simulink model "blown_lift_model"  (R2018b)
settings: Solver=ode45  StartTime=0.0  StopTime=100  RelTol=1e-5
model workspace (MAT data in the model file):
  aeroCoeff.CD = [0.115; 0.079; 0.047; 0.031; 0.027; 0.027; 0.029; 0.034; 0.054; 0.089]
  aeroCoeff.CL = [-1.421; -1.092; -0.695; -0.312; -0.132; 0.041; 0.218; 0.402; 0.786; 1.186]
  aeroCoeff.CM = [0.0775; 0.0663; 0.053; 0.0337; 0.0217; 0.0073; -0.009; -0.0263; -0.0632; -0.1235]
  aeroCoeff.CD_el = [0.0046  0.0029  0  -0.0009  -0.0008; 0.0039  0.0024  0  -0.0005  -0.0001; 0.0034  0.002  0  0  0.0005; 0.0028  0.0016  0  0.0004  0.0011; 0.0025  0.0014  0  0.0006  0.0014; 0.0022  0.0012  0  0.0008  0.0016; 0.0019  0.001  0  0.001  0.0019; 0.0016  0.0008  0  0.0012  0.0022; 0.001  0.0003  0  0.0016  0.0028; 0.0004  -0.0001  0  0.0021  0.0034]
  aeroCoeff.CL_el = [-0.051; -0.038; 0; 0.038; 0.052]
  aeroCoeff.CM_el = [0.0842; 0.0601; -0.0001; -0.0601; -0.0843]
  aeroCoeff.Xcp = [-0.055; -0.061; -0.076; -0.108; -0.164; 0.177; -0.041; -0.065; -0.08; -0.105]
  aeroCoeff.Mach_vec = [0.1 0.2 0.3 0.35]
  aeroCoeff.alpha_vec = [-16 -12 -8 -4 -2 0 2 4 8 12]
  aeroCoeff.def_vec = [-20 -10 0 10 20]
  environment.T0 = 275.15
  environment.a = 332.529
  environment.P0 = 79495.2
  environment.rho0 = 1.00649
  environment.vel_wind = [-2; 0; -0.1]
  environment.omega_wind = [0; 0; 0]
  environment.grav = [0 0 9.80665]
  initCond.alt0 = 2000
  initCond.x0 = [0 -2000]
  initCond.v0 = 93.1048
  initCond.alpha0 = 0.017092
  initCond.theta0 = 0.017092
  initCond.q0 = 0
  vehicle.Sref = 20.9775
  vehicle.cbar = 1.7526
  vehicle.bref = 12.54
  vehicle.CG = [0 0 0]
  vehicle.inertia_yy = 6928.93
  vehicle.acMass = 1299.214
  vehicle.Thrust = 2512.574
  vehicle.elevator_max = 20
  vehicle.elevator_min = -20
libraries: aerolibasang x3, shared3dof x1, sharedtransform x1
settings Model: Creator=Jacob  LastModifiedBy=william
settings SolverCC: MinimalZcImpactIntegration=on
settings DataIOCC: SaveFormat=Array
settings OptimizationCC: EnhancedBackFolding=on  StrengthReduction=on  InitFltsAndDblsToZero=on  DifferentSizesBufferReuse=on
settings DebuggingCC: WriteAfterWriteMsg=DisableAll  AlgebraicLoopMsg=none  FcnCallInpInsideContextMsg=warning  UnconnectedInputMsg=none  UnconnectedOutputMsg=none  UnconnectedLineMsg=none  UniqueDataStoreMsg=error  StateNameClashWarn=warning  LibraryContextMissingDiagnostic=none  StrictBusMsg=ErrorOnBusTreatedAsVector  SFUnexpectedBacktrackingDiag=warning  SFNoUnconditionalDefaultTransitionDiag=warning  SFExecutionAtInitializationDiag=none
settings ModelReferenceCC: PropagateSignalLabelsOutOfModel=off
settings SFSimCC: SimUseLocalCustomCode=off
settings RTWCC: RTWUseLocalCustomCode=off
settings CodeAppCC: StateflowObjectComments=on

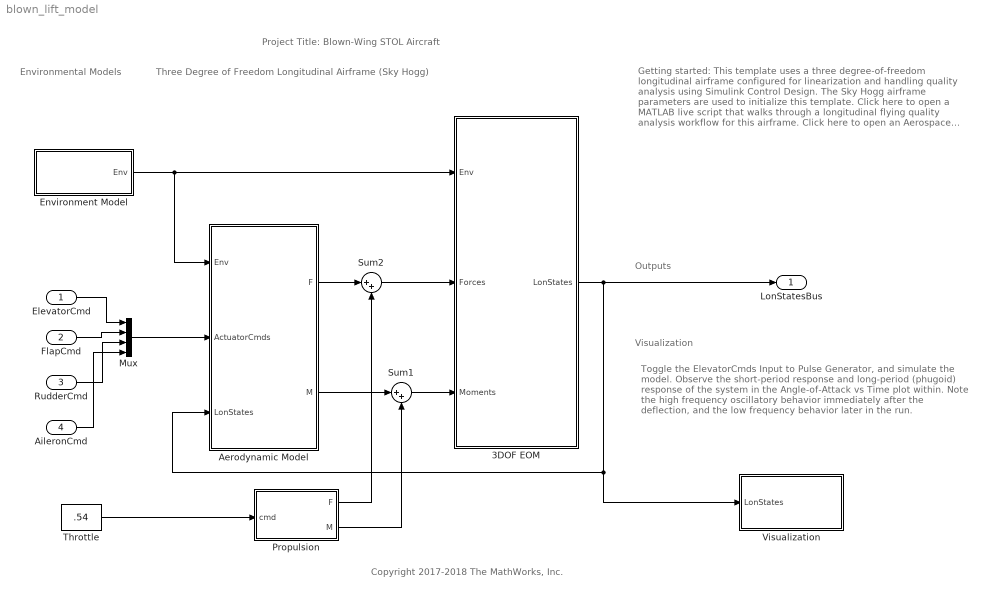
== system blown_lift_model ==
  note: Project Title: Blown-Wing STOL Aircraft
  note: Copyright 2017-2018 The MathWorks, Inc.
  note: Three Degree of Freedom Longitudinal Airframe (Sky Hogg)
  note: Environmental Models
  note: Toggle the ElevatorCmds Input to Pulse Generator, and simulate the model. Observe the short-period response and long-period (phugoid) response of the system in the Angle-of-Attack vs Time plot within. Note the high frequency oscillatory behavior immediately after the deflection, and the low frequency behavior later in the run.
  note: Visualization
  note: Outputs
  note: Getting started:
      | This template uses a three degree-of-freedom longitudinal airframe configured for linearization and handling quality analysis using Simulink Control Design. The Sky Hogg airframe parameters are used to initialize this template.
      |
      | Click here to open a MATLAB live script that walks through a longitudinal flying quality analysis workflow for this airframe.
      |
      | Click here to open an Aerospace Blockset Flight Control Analysis template that can be customized to perform flying quality analysis on your airframe model.
  ElevatorCmd : Inport
  FlapCmd : Inport  Port=2
  RudderCmd : Inport  Port=3
  AileronCmd : Inport  Port=4
  3DOF EOM : Subsystem  VariantControl=eom3DOF
  Aerodynamic Model : Subsystem  VariantControl=aeroCONST
  Environment Model : Subsystem  mask(Constant Environment Model){To=environment.T0, a=environment.a, Po=environment.P0, AirDensity=environment.rho0, ugvgwg=environment.vel_wind, pgqgrg=environment.omega_wind, g=environment.grav}
      mask prompts: To "Constant Temperature (K):"; a "Constant Speed of Sound (m/s):"; Po "Constant Pressure (Pa):"; AirDensity "Constant Air Density (kg/m^3):"; ugvgwg "Constant Wind Velocity [ug vg wg] (m/s):"; pgqgrg "Constant Wind Angular Rates [pg qg rg] (rad/s):"; g "Constant Gravitational Acceleration (m/s^2):"
      mask Help: helpview(fullfile(docroot,'toolbox','aeroblks','aeroblks.map'), 'environment1');
      mask TypeOptions To: Constant Atmosphere/To
      mask TypeOptions a: Constant Atmosphere/a
      mask TypeOptions Po: Constant Atmosphere/Po
      mask TypeOptions AirDensity: Constant Atmosphere/AirDensity
      mask TypeOptions ugvgwg: Constant Wind/ugvgwg
      mask TypeOptions pgqgrg: Constant Wind/pgqgrg
      mask TypeOptions g: Constant Gravity/g
      mask DialogControl Container4 Prompt: Atmospheric Model
      mask DialogControl Container6 Prompt: Wind Model
      mask DialogControl Container8 Prompt: Gravity Model
      mask Display:
      | image('aeroenvironment.bmp','center')
      | port_label('output',1,'Env')
  Mux : Mux
  Propulsion : Subsystem
      settings: RTWSystemCode=Inline
  Sum1 : Sum  Inputs=|++  SaturateOnIntegerOverflow=on  InputSameDT=on  OutDataTypeStr=Inherit: Same as first input
  Sum2 : Sum  Inputs=|++  SaturateOnIntegerOverflow=on  InputSameDT=on  OutDataTypeStr=Inherit: Same as first input
  Throttle : Constant  Value=.54
  Visualization : Subsystem
  LonStatesBus : Outport
  wires:
  3DOF EOM/1(LonStates) -> LonStatesBus/1, Visualization/1(LonStates), Aerodynamic Model/3(LonStates)
  Sum2/1 -> 3DOF EOM/2(Forces)
  Propulsion/2(M) -> Sum1/2
  Propulsion/1(F) -> Sum2/2
  Throttle/1 -> Propulsion/1(cmd)
  Sum1/1 -> 3DOF EOM/3(Moments)
  Aerodynamic Model/1(F) -> Sum2/1
  Aerodynamic Model/2(" M") -> Sum1/1
  Environment Model/1(Env) -> 3DOF EOM/1(Env), Aerodynamic Model/1(Env)
  ElevatorCmd/1 -> Mux/1
  FlapCmd/1 -> Mux/2
  RudderCmd/1 -> Mux/3
  AileronCmd/1 -> Mux/4
  Mux/1 -> Aerodynamic Model/2(ActuatorCmds)

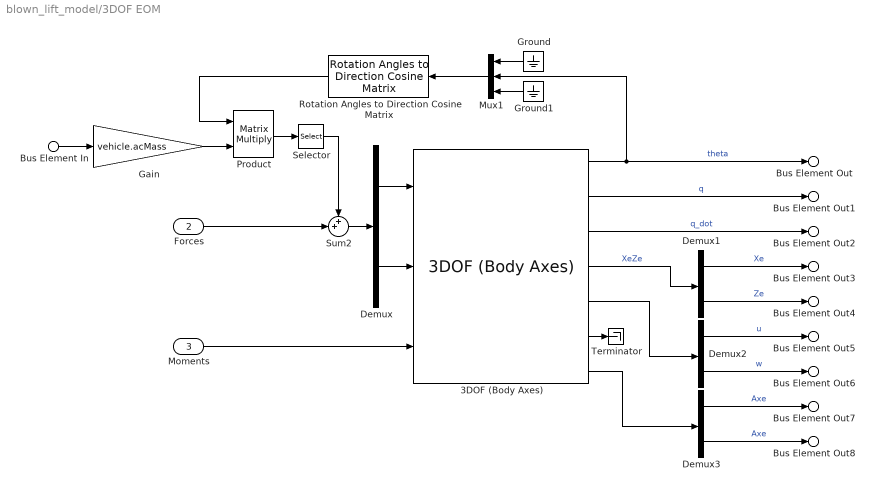
== system blown_lift_model/3DOF EOM ==
  Bus Element In : Inport  PortName=Env  Element=g
  Forces : Inport  Port=2
  Moments : Inport  Port=3
  3DOF (Body Axes) : shared3dof/3DOF (Body Axes)  units=Metric (MKS)  mtype=Fixed  v_ini=initCond.v0  theta_ini=initCond.theta0  alpha_ini=initCond.alpha0  pos_ini=initCond.x0  q_ini=initCond.q0  mass=vehicle.acMass  mass_e=0.5  mass_f=3.0  Iyy=vehicle.inertia_yy  Iyy_e=0.5  Iyy_f=3.0  g_in=Internal  g=0  vre_flag=on  abi_flag=on  aMode=0  vel_statename={'u', 'w'}  theta_statename='theta'  pos_statename={'Xe', 'Ze'}  q_statename='q'  mass_statename=''
      settings: SourceProductName=Aerospace Blockset  SourceProductBaseCode=AE
  Demux{,1..3} (4 alike) : Demux  Outputs=2
  Gain : Gain  Gain=vehicle.acMass
  Ground : Ground
  Ground1 : Ground
  Mux1 : Mux  Inputs=3
  Product : Product  Multiplication=Matrix(*)
  Rotation Angles to Direction Cosine Matrix : sharedtransform/Rotation Angles to Direction Cosine Matrix  rotationOrder=ZYX  aMode=aMode
      settings: SourceProductBaseCode=AE
  Selector : Selector  InputPortWidth=3  IndexOptions=Index vector (dialog)  Indices=[1 3]  OutputSizes=1
  Sum2 : Sum  Inputs=++|  SaturateOnIntegerOverflow=on  InputSameDT=on  OutDataTypeStr=Inherit: Same as first input
  Terminator : Terminator
  Bus Element Out : Outport  PortName=LonStates  Element=theta
  Bus Element Out1 : Outport  PortName=LonStates  Element=q
  Bus Element Out2 : Outport  PortName=LonStates  Element=q_dot
  Bus Element Out3 : Outport  PortName=LonStates  Element=Xe
  Bus Element Out4 : Outport  PortName=LonStates  Element=Ze
  Bus Element Out5 : Outport  PortName=LonStates  Element=u
  Bus Element Out6 : Outport  PortName=LonStates  Element=w
  Bus Element Out7 : Outport  PortName=LonStates  Element=Axe
  Bus Element Out8 : Outport  PortName=LonStates  Element=Aze
  wires:
  Demux/2 -> 3DOF (Body Axes)/2
  Demux/1 -> 3DOF (Body Axes)/1
  Sum2/1 -> Demux/1
  Selector/1 -> Sum2/1
  Ground1/1 -> Mux1/3
  Ground/1 -> Mux1/1
  Mux1/1 -> Rotation Angles to Direction Cosine Matrix/1
  Gain/1 -> Product/2
  Rotation Angles to Direction Cosine Matrix/1 -> Product/1
  Product/1 -> Selector/1
  Forces/1 -> Sum2/2
  Bus Element In/1 -> Gain/1
  Moments/1 -> 3DOF (Body Axes)/3
  3DOF (Body Axes)/1 -> Mux1/2, Bus Element Out/1  "theta"
  3DOF (Body Axes)/2 -> Bus Element Out1/1  "q"
  3DOF (Body Axes)/3 -> Bus Element Out2/1  "q_dot"
  3DOF (Body Axes)/4 -> Demux1/1  "XeZe"
  3DOF (Body Axes)/5 -> Demux2/1
  3DOF (Body Axes)/7 -> Demux3/1
  Demux3/1 -> Bus Element Out7/1  "Axe"
  Demux3/2 -> Bus Element Out8/1  "Axe"
  Demux2/2 -> Bus Element Out6/1  "w"
  Demux2/1 -> Bus Element Out5/1  "u"
  Demux1/2 -> Bus Element Out4/1  "Ze"
  Demux1/1 -> Bus Element Out3/1  "Xe"
  3DOF (Body Axes)/6 -> Terminator/1

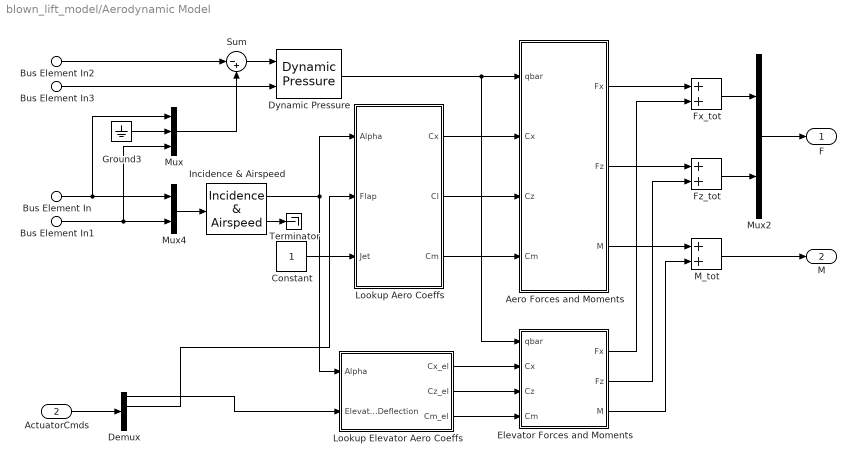
== system blown_lift_model/Aerodynamic Model ==
  Bus Element In2 : Inport  PortName=Env  Element=WindVelocity
  Bus Element In3 : Inport  PortName=Env  Element=AirDensity
  ActuatorCmds : Inport  Port=2
  Bus Element In : Inport  Port=3  PortName=LonStates  Element=u
  Bus Element In1 : Inport  Port=3  PortName=LonStates  Element=w
  Aero Forces and Moments : Subsystem
  Constant : Constant
  Demux : Demux
  Dynamic Pressure : aerolibasang/Dynamic Pressure
  Elevator Forces and Moments : Subsystem
  Fx_tot : Sum  SaturateOnIntegerOverflow=on  InputSameDT=on  OutDataTypeStr=Inherit: Same as first input
  Fz_tot : Sum  SaturateOnIntegerOverflow=on  InputSameDT=on  OutDataTypeStr=Inherit: Same as first input
  Ground3 : Ground
  Incidence & Airspeed : aerolibasang/Incidence  & Airspeed
      settings: SourceProductName=Aerospace Blockset  SourceProductBaseCode=AE
  Lookup Aero Coeffs : Subsystem
  Lookup Elevator Aero Coeffs : Subsystem
  M_tot : Sum  SaturateOnIntegerOverflow=on  InputSameDT=on  OutDataTypeStr=Inherit: Same as first input
  Mux : Mux  Inputs=3
  Mux2 : Mux  Inputs=2
  Mux4 : Mux  Inputs=2
  Sum : Sum  Inputs=|-+
  Terminator : Terminator
  F : Outport
  " M" : Outport  Port=2  Unit=N*m
  wires:
  Bus Element In3/1 -> Dynamic Pressure/2
  Bus Element In2/1 -> Sum/1
  Incidence & Airspeed/2 -> Terminator/1
  Bus Element In/1 -> Mux4/1, Mux/1
  Bus Element In1/1 -> Mux4/2, Mux/3
  Mux2/1 -> F/1
  Mux4/1 -> Incidence & Airspeed/1
  Ground3/1 -> Mux/2
  M_tot/1 -> " M"/1
  Sum/1 -> Dynamic Pressure/1
  Incidence & Airspeed/1 -> Lookup Aero Coeffs/1(Alpha), Lookup Elevator Aero Coeffs/1(Alpha)
  Mux/1 -> Sum/2
  Elevator Forces and Moments/3(M) -> M_tot/2
  Dynamic Pressure/1 -> Elevator Forces and Moments/1(qbar), Aero Forces and Moments/1(qbar)
  Aero Forces and Moments/1(Fx) -> Fx_tot/1
  Aero Forces and Moments/3(M) -> M_tot/1
  Lookup Aero Coeffs/1(Cx) -> Aero Forces and Moments/2(Cx)
  Lookup Aero Coeffs/2(Cl) -> Aero Forces and Moments/3(Cz)
  Lookup Aero Coeffs/3(Cm) -> Aero Forces and Moments/4(Cm)
  Lookup Elevator Aero Coeffs/1(Cx_el) -> Elevator Forces and Moments/2(Cx)
  Lookup Elevator Aero Coeffs/2(Cz_el) -> Elevator Forces and Moments/3(Cz)
  Lookup Elevator Aero Coeffs/3(Cm_el) -> Elevator Forces and Moments/4(Cm)
  Elevator Forces and Moments/1(Fx) -> Fx_tot/2
  Elevator Forces and Moments/2(Fz) -> Fz_tot/2
  Aero Forces and Moments/2(Fz) -> Fz_tot/1
  Fx_tot/1 -> Mux2/1
  Fz_tot/1 -> Mux2/2
  ActuatorCmds/1 -> Demux/1
  Demux/1 -> Lookup Elevator Aero Coeffs/2(Elevator Deflection)
  Demux/2 -> Lookup Aero Coeffs/2(Flap)
  Constant/1 -> Lookup Aero Coeffs/3(Jet)

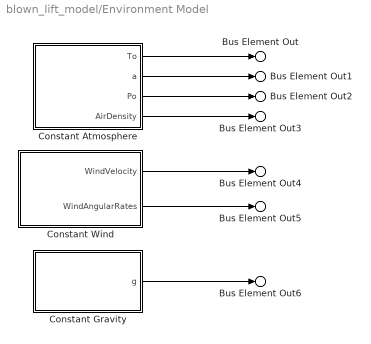
== system blown_lift_model/Environment Model ==
  Constant Atmosphere : Subsystem  VariantControl=atmosCONST  mask(Standard Atmospheric Constants){To=To, a=a, Po=Po, AirDensity=AirDensity}
      mask prompts: To "Constant Temperature (K):"; a "Constant Speed of Sound (m/s):"; Po "Constant Pressure (Pa):"; AirDensity "Constant Air Density (kg/m^3):"
  Constant Gravity : Subsystem  VariantControl=gravCONST  mask(Constant Gravitational Acceleration){g=g}
      mask prompts: g "Constant Gravitational Acceleration (m/s^2):"
  Constant Wind : Subsystem  VariantControl=windCONST  mask(Constant Wind Values){ugvgwg=ugvgwg, pgqgrg=pgqgrg}
      mask prompts: ugvgwg "Constant Wind Velocity (m/s):"; pgqgrg "Constant Wind Angular Rates (rad/s):"
  Bus Element Out : Outport  PortName=Env  Element=To
  Bus Element Out1 : Outport  PortName=Env  Element=a
  Bus Element Out2 : Outport  PortName=Env  Element=Po
  Bus Element Out3 : Outport  PortName=Env  Element=AirDensity
  Bus Element Out4 : Outport  PortName=Env  Element=WindVelocity
  Bus Element Out5 : Outport  PortName=Env  Element=WindAngularRates
  Bus Element Out6 : Outport  PortName=Env  Element=g
  wires:
  Constant Wind/2(WindAngularRates) -> Bus Element Out5/1
  Constant Atmosphere/3(Po) -> Bus Element Out2/1
  Constant Atmosphere/4(AirDensity) -> Bus Element Out3/1
  Constant Atmosphere/1(To) -> Bus Element Out/1
  Constant Wind/1(WindVelocity) -> Bus Element Out4/1
  Constant Atmosphere/2(a) -> Bus Element Out1/1
  Constant Gravity/1(g) -> Bus Element Out6/1

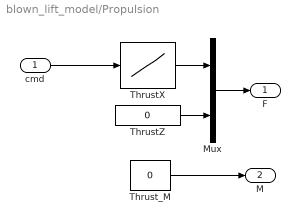
== system blown_lift_model/Propulsion ==
  cmd : Inport
  Mux : Mux  Inputs=2
  ThrustX : Lookup_n-D  NumberOfTableDimensions=1  LookupTableObject=''  BreakpointsForDimension1=(1/6)*(3+([-3:3]))  IndexSearchMethod=Linear search  BeginIndexSearchUsingPreviousIndexResult=on  Table=vehicle.Thrust*(1+tanh([-3:3]))  ExtrapMethod=Clip  InputSameDT=on
  ThrustZ : Constant  Value=0  SampleTime=-1
  Thrust_M : Constant  Value=0  SampleTime=-1
  F : Outport  Unit=N
  M : Outport  Port=2  Unit=N*m
  wires:
  cmd/1 -> ThrustX/1
  Thrust_M/1 -> M/1
  Mux/1 -> F/1
  ThrustZ/1 -> Mux/2
  ThrustX/1 -> Mux/1

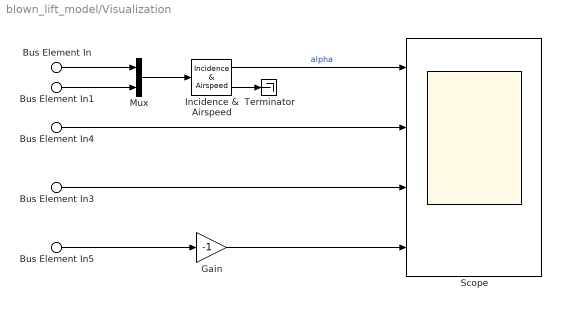
== system blown_lift_model/Visualization ==
  Bus Element In : Inport  PortName=LonStates  Element=u
  Bus Element In1 : Inport  PortName=LonStates  Element=w
  Bus Element In3 : Inport  PortName=LonStates  Element=q
  Bus Element In4 : Inport  PortName=LonStates  Element=theta
  Bus Element In5 : Inport  PortName=LonStates  Element=Ze
  Gain : Gain  Gain=-1
  Incidence & Airspeed : aerolibasang/Incidence  & Airspeed
      settings: SourceProductName=Aerospace Blockset  SourceProductBaseCode=AE
  Mux : Mux  Inputs=2
  Scope : Scope  NumInputPorts=4
  Terminator : Terminator
  wires:
  Gain/1 -> Scope/4
  Bus Element In5/1 -> Gain/1
  Bus Element In4/1 -> Scope/2
  Bus Element In3/1 -> Scope/3
  Mux/1 -> Incidence & Airspeed/1
  Bus Element In1/1 -> Mux/2
  Bus Element In/1 -> Mux/1
  Incidence & Airspeed/2 -> Terminator/1
  Incidence & Airspeed/1 -> Scope/1  "alpha"

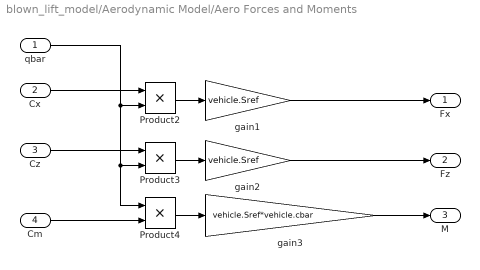
== system blown_lift_model/Aerodynamic Model/Aero Forces and Moments ==
  qbar : Inport
  Cx : Inport  Port=2
  Cz : Inport  Port=3
  Cm : Inport  Port=4
  Product2 : Product  SaturateOnIntegerOverflow=on  InputSameDT=on  OutDataTypeStr=Inherit: Same as first input
  Product3 : Product  SaturateOnIntegerOverflow=on  InputSameDT=on  OutDataTypeStr=Inherit: Same as first input
  Product4 : Product  SaturateOnIntegerOverflow=on  InputSameDT=on  OutDataTypeStr=Inherit: Same as first input
  gain1 : Gain  Gain=vehicle.Sref  SaturateOnIntegerOverflow=on  OutDataTypeStr=Inherit: Same as input  ParamDataTypeStr=Inherit: Same as input
  "gain2 " : Gain  Gain=vehicle.Sref  SaturateOnIntegerOverflow=on  OutDataTypeStr=Inherit: Same as input  ParamDataTypeStr=Inherit: Same as input
  gain3 : Gain  Gain=vehicle.Sref*vehicle.cbar  SaturateOnIntegerOverflow=on  OutDataTypeStr=Inherit: Same as input  ParamDataTypeStr=Inherit: Same as input
  Fx : Outport
  Fz : Outport  Port=2
  M : Outport  Port=3
  wires:
  gain3/1 -> M/1
  "gain2 "/1 -> Fz/1
  qbar/1 -> Product2/2, Product4/1, Product3/2
  Product4/1 -> gain3/1
  Product2/1 -> gain1/1
  Cm/1 -> Product4/2
  Product3/1 -> "gain2 "/1
  Cz/1 -> Product3/1
  Cx/1 -> Product2/1
  gain1/1 -> Fx/1

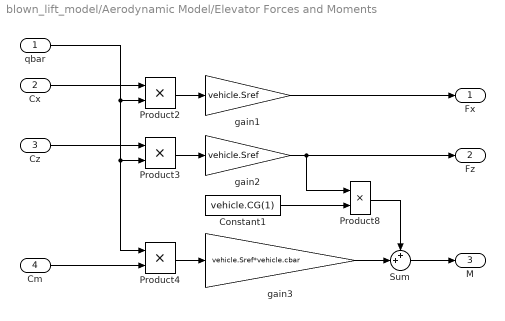
== system blown_lift_model/Aerodynamic Model/Elevator Forces and Moments ==
  qbar : Inport
  Cx : Inport  Port=2
  Cz : Inport  Port=3
  Cm : Inport  Port=4
  Constant1 : Constant  Value=vehicle.CG(1)
  Product2 : Product  SaturateOnIntegerOverflow=on  InputSameDT=on  OutDataTypeStr=Inherit: Same as first input
  Product3 : Product  SaturateOnIntegerOverflow=on  InputSameDT=on  OutDataTypeStr=Inherit: Same as first input
  Product4 : Product  SaturateOnIntegerOverflow=on  InputSameDT=on  OutDataTypeStr=Inherit: Same as first input
  Product8 : Product
  Sum : Sum  Inputs=++|
  gain1 : Gain  Gain=vehicle.Sref  SaturateOnIntegerOverflow=on  OutDataTypeStr=Inherit: Same as input  ParamDataTypeStr=Inherit: Same as input
  "gain2 " : Gain  Gain=vehicle.Sref  SaturateOnIntegerOverflow=on  OutDataTypeStr=Inherit: Same as input  ParamDataTypeStr=Inherit: Same as input
  gain3 : Gain  Gain=vehicle.Sref*vehicle.cbar  SaturateOnIntegerOverflow=on  OutDataTypeStr=Inherit: Same as input  ParamDataTypeStr=Inherit: Same as input
  Fx : Outport
  Fz : Outport  Port=2
  M : Outport  Port=3
  wires:
  Sum/1 -> M/1
  "gain2 "/1 -> Product8/1, Fz/1
  Constant1/1 -> Product8/2
  Product8/1 -> Sum/1
  gain3/1 -> Sum/2
  gain1/1 -> Fx/1
  Cx/1 -> Product2/1
  Cz/1 -> Product3/1
  Product3/1 -> "gain2 "/1
  Cm/1 -> Product4/2
  Product2/1 -> gain1/1
  Product4/1 -> gain3/1
  qbar/1 -> Product2/2, Product3/2, Product4/1

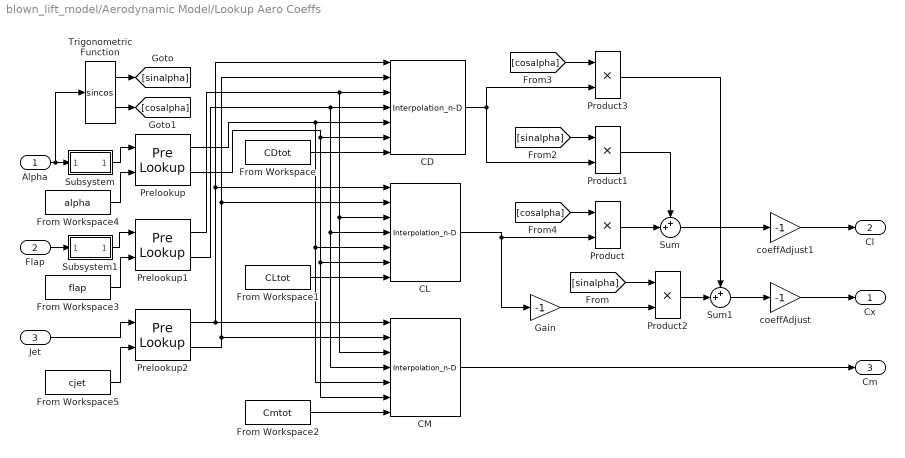
== system blown_lift_model/Aerodynamic Model/Lookup Aero Coeffs ==
  Alpha : Inport  Unit=rad
  Flap : Inport  Port=2  Unit=rad
  Jet : Inport  Port=3  Unit=rad
  CD : Interpolation_n-D  NumberOfTableDimensions=3  TableSource=Input port  Table=aeroCoeff.CD  LookupTableObject=CDtot  InternalRulePriority=Speed
      settings: InputPortMap=u0,u1,u2,u3,u4,u5,p2
  CL : Interpolation_n-D  NumberOfTableDimensions=3  TableSource=Input port  Table=[-1.421,-1.092,-0.695,-0.312,-0.132,0.041,0.218,0.402,0.786,1.186]  InternalRulePriority=Speed
      settings: InputPortMap=u0,u1,u2,u3,u4,u5,p2
  CM : Interpolation_n-D  NumberOfTableDimensions=3  TableSource=Input port  Table=aeroCoeff.CM  InternalRulePriority=Speed
      settings: InputPortMap=u0,u1,u2,u3,u4,u5,p2
  From Workspace : FromWorkspace  VariableName=CDtot
  From Workspace1 : FromWorkspace  VariableName=CLtot  SampleTime=0
  From Workspace2 : FromWorkspace  VariableName=Cmtot  SampleTime=0
  From Workspace3 : FromWorkspace  VariableName=flap
  From Workspace4 : FromWorkspace  VariableName=alpha
  From Workspace5 : FromWorkspace  VariableName=cjet  SampleTime=0
  Gain : Gain  Gain=-1
  Prelookup : PreLookup  BreakpointsDataSource=Input port  BreakpointsData=aeroCoeff.alpha_vec  ExtrapMethod=Linear
      settings: InputPortMap=u0,p1
  Prelookup1 : PreLookup  BreakpointsDataSource=Input port  BreakpointsData=aeroCoeff.alpha_vec  ExtrapMethod=Linear
      settings: InputPortMap=u0,p1
  Prelookup2 : PreLookup  BreakpointsDataSource=Input port  BreakpointsData=aeroCoeff.alpha_vec  ExtrapMethod=Linear
      settings: InputPortMap=u0,p1
  Product{,1..3} (4 alike) : Product
  Subsystem : Subsystem
      mask Display:
      | port_label('output',1,'deg')
      | port_label('input',1,'rad')
  Subsystem1 : Subsystem
      mask Display:
      | port_label('output',1,'deg')
      | port_label('input',1,'rad')
  Sum : Sum  Inputs=++|
  Sum1 : Sum  Inputs=++|
  Trigonometric Function : Trigonometry  Operator=sincos
  coeffAdjust : Gain  Gain=-1
  coeffAdjust1 : Gain  Gain=-1
  Cx : Outport
  Cl : Outport  Port=2
  Cm : Outport  Port=3
  wires:
  Subsystem/1(Out2) -> Prelookup/1
  Trigonometric Function/1 -> [sinalpha]
  Trigonometric Function/2 -> [cosalpha]
  [cosalpha] -> Product/1
  [cosalpha] -> Product3/1
  [sinalpha] -> Product1/1
  [sinalpha] -> Product2/1
  Alpha/1 -> Trigonometric Function/1, Subsystem/1(In1)
  coeffAdjust/1 -> Cx/1
  coeffAdjust1/1 -> Cl/1
  Sum1/1 -> coeffAdjust/1
  Product3/1 -> Sum1/1
  Product2/1 -> Sum1/2
  Gain/1 -> Product2/2
  Sum/1 -> coeffAdjust1/1
  Product1/1 -> Sum/1
  CD/1 -> Product1/2, Product3/2
  Product/1 -> Sum/2
  CM/1 -> Cm/1
  CL/1 -> Product/2, Gain/1
  From Workspace/1 -> CD/7
  From Workspace1/1 -> CL/7
  From Workspace2/1 -> CM/7
  Flap/1 -> Subsystem1/1(In1)
  Subsystem1/1(Out2) -> Prelookup1/1
  Prelookup1/1 -> CM/3, CL/3, CD/3
  Prelookup1/2 -> CM/4, CL/4, CD/4
  Jet/1 -> Prelookup2/1
  Prelookup/1 -> CM/5, CL/5, CD/5
  Prelookup/2 -> CM/6, CL/6, CD/6
  Prelookup2/1 -> CM/1, CL/1, CD/1
  Prelookup2/2 -> CM/2, CL/2, CD/2
  From Workspace5/1 -> Prelookup2/2
  From Workspace3/1 -> Prelookup1/2
  From Workspace4/1 -> Prelookup/2

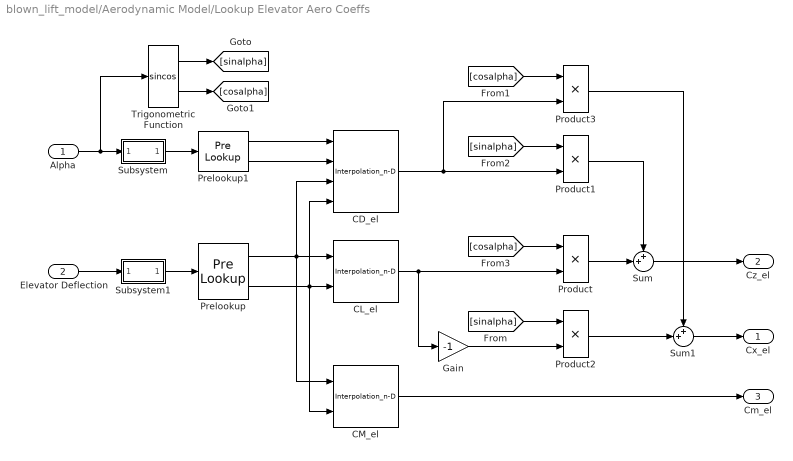
== system blown_lift_model/Aerodynamic Model/Lookup Elevator Aero Coeffs ==
  Alpha : Inport  Unit=rad
  Elevator Deflection : Inport  Port=2  Unit=rad
  CD_el : Interpolation_n-D  Table=aeroCoeff.CD_el
  CL_el : Interpolation_n-D  NumberOfTableDimensions=1  Table=aeroCoeff.CL_el  InternalRulePriority=Speed
      settings: InputPortMap=u0,u1
  CM_el : Interpolation_n-D  NumberOfTableDimensions=1  Table=aeroCoeff.CM_el  InternalRulePriority=Speed
      settings: InputPortMap=u0,u1
  Gain : Gain  Gain=-1
  Prelookup : PreLookup  BreakpointsData=aeroCoeff.def_vec  ExtrapMethod=Linear  IndexDataTypeStr=int32  FractionDataTypeStr=double
  Prelookup1 : PreLookup  BreakpointsData=aeroCoeff.alpha_vec  ExtrapMethod=Linear  IndexDataTypeStr=int32  FractionDataTypeStr=double
  Product{,1..3} (4 alike) : Product
  Subsystem : Subsystem
      mask Display:
      | port_label('output',1,'deg')
      | port_label('input',1,'rad')
  Subsystem1 : Subsystem
      mask Display:
      | port_label('output',1,'deg')
      | port_label('input',1,'rad')
  Sum : Sum  Inputs=++|
  Sum1 : Sum  Inputs=++|
  Trigonometric Function : Trigonometry  Operator=sincos
  Cx_el : Outport
  Cz_el : Outport  Port=2
  Cm_el : Outport  Port=3
  wires:
  Subsystem1/1(Out2) -> Prelookup/1
  Trigonometric Function/1 -> [sinalpha]
  Trigonometric Function/2 -> [cosalpha]
  [cosalpha] -> Product/1
  [cosalpha] -> Product3/1
  [sinalpha] -> Product1/1
  [sinalpha] -> Product2/1
  Prelookup1/2 -> CD_el/2
  Prelookup1/1 -> CD_el/1
  Elevator Deflection/1 -> Subsystem1/1(In1)
  Subsystem/1(Out2) -> Prelookup1/1
  Alpha/1 -> Trigonometric Function/1, Subsystem/1(In1)
  Prelookup/2 -> CM_el/2, CL_el/2, CD_el/4
  Prelookup/1 -> CD_el/3, CL_el/1, CM_el/1
  CD_el/1 -> Product3/2, Product1/2
  Gain/1 -> Product2/2
  Product3/1 -> Sum1/1
  CL_el/1 -> Gain/1, Product/2
  Product2/1 -> Sum1/2
  Product/1 -> Sum/2
  Product1/1 -> Sum/1
  Sum/1 -> Cz_el/1
  CM_el/1 -> Cm_el/1
  Sum1/1 -> Cx_el/1

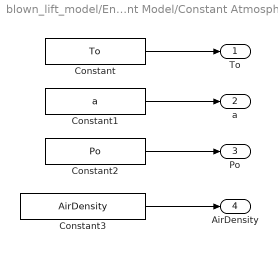
== system blown_lift_model/Environment Model/Constant Atmosphere ==
  Constant : Constant  Value=To
  Constant1 : Constant  Value=a
  Constant2 : Constant  Value=Po
  Constant3 : Constant  Value=AirDensity
  To : Outport
  a : Outport  Port=2
  Po : Outport  Port=3
  AirDensity : Outport  Port=4
  wires:
  Constant1/1 -> a/1
  Constant/1 -> To/1
  Constant2/1 -> Po/1
  Constant3/1 -> AirDensity/1

== system blown_lift_model/Environment Model/Constant Gravity ==
  Reshape1 : Reshape  OutputDimensionality=Column vector (2-D)
  Standard Gravity : Constant  Value=g
  g : Outport
  wires:
  Reshape1/1 -> g/1
  Standard Gravity/1 -> Reshape1/1

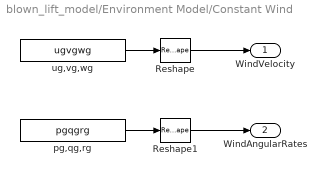
== system blown_lift_model/Environment Model/Constant Wind ==
  Reshape : Reshape  OutputDimensionality=Column vector (2-D)
  Reshape1 : Reshape  OutputDimensionality=Column vector (2-D)
  pg,qg,rg : Constant  Value=pgqgrg
  ug,vg,wg : Constant  Value=ugvgwg
  WindVelocity : Outport
  WindAngularRates : Outport  Port=2
  wires:
  pg,qg,rg/1 -> Reshape1/1
  ug,vg,wg/1 -> Reshape/1
  Reshape/1 -> WindVelocity/1
  Reshape1/1 -> WindAngularRates/1

== system blown_lift_model/Aerodynamic Model/Lookup Aero Coeffs/Subsystem ==
  In1 : Inport
  Signal Specification : SignalSpecification  Unit=deg
  Unit Conversion : UnitConversion
  Out2 : Outport
  wires:
  In1/1 -> Unit Conversion/1
  Unit Conversion/1 -> Signal Specification/1
  Signal Specification/1 -> Out2/1

== system blown_lift_model/Aerodynamic Model/Lookup Aero Coeffs/Subsystem1 ==
  In1 : Inport
  Signal Specification : SignalSpecification  Unit=deg
  Unit Conversion : UnitConversion
  Out2 : Outport
  wires:
  In1/1 -> Unit Conversion/1
  Unit Conversion/1 -> Signal Specification/1
  Signal Specification/1 -> Out2/1

== system blown_lift_model/Aerodynamic Model/Lookup Elevator Aero Coeffs/Subsystem ==
  In1 : Inport
  Signal Specification : SignalSpecification  Unit=deg
  Unit Conversion : UnitConversion
  Out2 : Outport
  wires:
  In1/1 -> Unit Conversion/1
  Unit Conversion/1 -> Signal Specification/1
  Signal Specification/1 -> Out2/1

== system blown_lift_model/Aerodynamic Model/Lookup Elevator Aero Coeffs/Subsystem1 ==
  In1 : Inport
  Signal Specification : SignalSpecification  Unit=deg
  Unit Conversion : UnitConversion
  Out2 : Outport
  wires:
  Signal Specification/1 -> Out2/1
  Unit Conversion/1 -> Signal Specification/1
  In1/1 -> Unit Conversion/1
